simulink model "usrp_4t12r_heatmap"  (R2018a)
settings: Solver=VariableStepDiscrete  StartTime=0.0  StopTime=inf  RelTol=1e-3
undefined symbols (not defined in the file): fft2, gather, get, gpuArray, parula, psBcoor, psWcen, rfcaptureC2Fsim, Time, tsRamp, us
libraries: neural x14, visionanalysis x8, dspobslib x8, dspfdesign x7, dspstat3 x5, dspbuff3 x2, visionsinks x2, commsdrhw_v2 x1, visiontextngfix x1, dspvision x1, visiontransforms x1, dspsigops x1
(part 2 of 4)

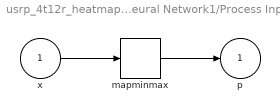
== system usrp_4t12r_heatmap/定位系统/定位模块/Pattern Recognition Neural Network1/Process Input 1 ==
  x : Inport  PortDimensions=627
      mask Display: e = 0.06;c1 = [120 230 180]/255;c2 = ([120 230 180]+0)/(256+128);c3 = ([120 230 180]+128)/(256+128);patch([0 1 1 0],[0 0 1 1],c1);patch([0 1 1 1-e 1-e 0+e],[0 0 1 1-e 0+e 0+e],c2);patch([0 0 1 1-e 0+e 0+e],[0 1 1 1-e 1-e 0+e],c3);plot([0 1 1 0 0],[0 0 1 1 0]);
  mapminmax : neural/Processing Functions/mapminmax  xmin=[0.183030532688018526821238651792;0.190861261961224687455640491862;0.194146917626080439678304401241;0.183721955574710132941262941131;0.201842690762400661652620215136;0.220412633155252224437248287359;0.210318465182484953812647177074;0.225823707454154809504132117581;0.243135323014785853512620406036;0.221810071164261130016726042413;0.218352813453565136603273799665;0.217860424693131021767200650174;0.211451016642378614163177985574;0.209356237294615388222496221715;0.205818369605545864464701821817;0.197728209339595090154872991661;0.190530847063016622877640315892;0.167795272037218085037224568623;0.144670324129353350395277288953;0.183030532688018526821238651792;0.190861261961224687455640491862;0.194146917626080439678304401241;0.183721955574710132941262941131;0.201842690762400661652620215136;0.220412633155252224437248287359;0.210318465182484953812647177074;0.225823707454154809504132117581;0.243135323014785853512620406036;0.221810071164261130016726042413;0.218352813453565136603273799665;0.217860424693131021767200650174;0.211451016642378614163177985574;0.209356237294615388222496221715;0.205818369605545864464701821817;0.197728209339595090154872991661;0.190530847063016622877640315892;0.167795272037218085037224568623;0.144670324129353350395277288953;0.183030532688018526821238651792;0.190861261961224687455640491862;0.194146917626080439678304401241;0.183721955574710132941262941131;0.201842690762400661652620215136;0.220412633155252224437248287359;0.210318465182484953812647177074;0.225823707454154809504132117581;0.243135323014785853512620406036;0.221810071164261130016726042413;0.218352813453565136603273799665;0.217860424693131021767200650174;0.211451016642378614163177985574;0.209356237294615388222496221715;0.205818369605545864464701821817;0.197728209339595090154872991661;0.190530847063016622877640315892;0.167795272037218085037224568623;0.144670324129353350395277288953;0.183030532688018526821238651792;0.190861261961224687455640491862;0.194146917626080439678304401241;0.183721955574710132941262941131;0.201842690762400661652620215136;0.220412633155252224437248287359;0.210318465182484953812647177074;0.225823707454154809504132117581;0.243135323014785853512620406036;0.221810071164261130016726042413;0.218352813453565136603273799665;0.217860424693131021767200650174;0.211451016642378614163177985574;0.209356237294615388222496221715;0.205818369605545864464701821817;0.197728209339595090154872991661;0.190530847063016622877640315892;0.167795272037218085037224568623;0.144670324129353350395277288953;0.188373791055123723792164014412;0.196433124862748803574064027089;0.194146917626080439678304401241;0.183721955574710132941262941131;0.201842690762400661652620215136;0.220412633155252224437248287359;0.210318465182484953812647177074;0.225823707454154809504132117581;0.243135323014785853512620406036;0.221810071164261130016726042413;0.218352813453565136603273799665;0.217860424693131021767200650174;0.211451016642378614163177985574;0.209356237294615388222496221715;0.205818369605545864464701821817;0.197728209339595090154872991661;0.190530847063016622877640315892;0.167795272037218085037224568623;0.144670324129353350395277288953;0.188373791055123723792164014412;0.196433124862748803574064027089;0.194146917626080439678304401241;0.183721955574710132941262941131;0.201842690762400661652620215136;0.220412633155252224437248287359;0.210318465182484953812647177074;0.225823707454154809504132117581;0.243135323014785853512620406036;0.221810071164261130016726042413;0.218352813453565136603273799665;0.217860424693131021767200650174;0.211451016642378614163177985574;0.209356237294615388222496221715;0.205818369605545864464701821817;0.197728209339595090154872991661;0.190530847063016622877640315892;0.167795272037218085037224568623;0.144670324129353350395277288953;0.197827438261914317907397276031;0.204571901720102755639629776852;0.194146917626080439678304401241;0.183721955574710132941262941131;0.201842690762400661652620215136;0.220412633155252224437248287359;0.216458347323125160910350928134 ...(+16650 chars)]  xmax=[1;0.957688668661197506359883391269;0.957956127733447404537514557887;1;0.996524641407459332853591149615;1;1;1;1;1;1;1;1;1;1;1;0.992949114404950594625631765666;0.983183728188606664843973703682;0.975467151452690028889946916024;1;0.960233553399059580613084108336;0.957956127733447404537514557887;1;0.996524641407459332853591149615;1;1;0.996308649645406885220211279375;1;1;1;0.99394380170718721334566225778;1;1;1;1;0.992949114404950594625631765666;0.983183728188606664843973703682;0.975467151452690028889946916024;1;0.960233553399059580613084108336;0.971339192350340052684032343677;1;0.996524641407459332853591149615;1;1;0.987208758234387806496101802622;0.996476557864772627404192917311;1;1;0.99394380170718721334566225778;1;1;0.996365674241340815164846844709;1;0.992949114404950594625631765666;0.983183728188606664843973703682;0.975467151452690028889946916024;1;0.960233553399059580613084108336;0.971339192350340052684032343677;1;1;1;1;0.987208758234387806496101802622;0.998269531990686354028241566994;1;1;0.99394380170718721334566225778;1;1;1;1;0.992949114404950594625631765666;0.983183728188606664843973703682;0.975467151452690028889946916024;0.992019539944344441728674155456;0.960233553399059580613084108336;0.971339192350340052684032343677;1;1;1;1;0.987208758234387806496101802622;0.998269531990686354028241566994;1;1;0.99394380170718721334566225778;1;1;1;1;0.992949114404950594625631765666;0.983183728188606664843973703682;0.975467151452690028889946916024;0.965464417572932775968297391955;0.952570447882058246591441275086;0.971339192350340052684032343677;1;1;1;1;0.976132306177093567178815192165;0.998269531990686354028241566994;1;0.984196482050718746137363268645;0.99394380170718721334566225778;1;1;1;1;0.992949114404950594625631765666;0.983183728188606664843973703682;0.975467151452690028889946916024;0.953175834974080649075744986476;0.932443563986340873128710882156;0.971339192350340052684032343677;1;1;1;1;0.976132306177093567178815192165;0.998269531990686354028241566994;1;0.984196482050718746137363268645;0.99394380170718721334566225778;1;1;1;1;0.992949114404950594625631765666;0.983183728188606664843973703682;0.975467151452690028889946916024;0.981027149358607908347096326906;1;0.978869445923384651209175899567;0.991702730309424129728768093628;1;1;1;0.980384429143986713128811061324;0.998269531990686354028241566994;1;0.984196482050718746137363268645;0.99394380170718721334566225778;1;1;1;1;0.992949114404950594625631765666;0.983183728188606664843973703682;0.975467151452690028889946916024;0.981027149358607908347096326906;1;0.978869445923384651209175899567;0.991702730309424129728768093628;1;1;1;0.980384429143986713128811061324;0.998269531990686354028241566994;1;0.984196482050718746137363268645;0.99394380170718721334566225778;1;1;1;1;0.992949114404950594625631765666;0.983183728188606664843973703682;0.975467151452690028889946916024;0.981027149358607908347096326906;1;0.978869445923384651209175899567;0.991702730309424129728768093628;1;1;1;0.980384429143986713128811061324;0.998269531990686354028241566994;1;0.984196482050718746137363268645;0.99394380170718721334566225778;1;1;1;1;0.992949114404950594625631765666;0.983183728188606664843973703682;0.975467151452690028889946916024;0.981027149358607908347096326906;1;0.978869445923384651209175899567;0.991702730309424129728768093628;1;1;1;0.980384429143986713128811061324;0.998269531990686354028241566994;1;0.984196482050718746137363268645;0.99394380170718721334566225778;1;1;1;1;0.992949114404950594625631765666;0.983183728188606664843973703682;0.975467151452690028889946916024;0.981027149358607908347096326906;1;0.978869445923384651209175899567;0.991702730309424129728768093628;1;1;1;0.980384429143986713128811061324;0.998269531990686354028241566994;1;0.998970019032386580271065668057;1;1;1;1;0.999424539007601864248897527432;0.992949114404950594625631765666;0.983183728188606664843973703682;0.975467151452690028889946916024;0.981027149358607908347096326906;1;0.978869445923384651209175899567;0.991702730309424129728768093628;1;1;1 ...(+8309 chars)]  ymin=-1  ymax=1
  p : Outport  PortDimensions=627
      mask Display: e = 0.06;c1 = [120 230 180]/255;c2 = ([120 230 180]+0)/(256+128);c3 = ([120 230 180]+128)/(256+128);patch([0 1 1 0],[0 0 1 1],c1);patch([0 1 1 1-e 1-e 0+e],[0 0 1 1-e 0+e 0+e],c2);patch([0 0 1 1-e 0+e 0+e],[0 1 1 1-e 1-e 0+e],c3);plot([0 1 1 0 0],[0 0 1 1 0]);
  wires:
  x/1 -> mapminmax/1
  mapminmax/1 -> p/1

== system usrp_4t12r_heatmap/定位系统/定位模块/Pattern Recognition Neural Network1/Process Output 1 ==
  a : Inport  PortDimensions=1
      mask Display: e = 0.06;c1 = [120 230 180]/255;c2 = ([120 230 180]+0)/(256+128);c3 = ([120 230 180]+128)/(256+128);patch([0 1 1 0],[0 0 1 1],c1);patch([0 1 1 1-e 1-e 0+e],[0 0 1 1-e 0+e 0+e],c2);patch([0 0 1 1-e 0+e 0+e],[0 1 1 1-e 1-e 0+e],c3);plot([0 1 1 0 0],[0 0 1 1 0]);
  y : Outport  PortDimensions=1
      mask Display: e = 0.06;c1 = [120 230 180]/255;c2 = ([120 230 180]+0)/(256+128);c3 = ([120 230 180]+128)/(256+128);patch([0 1 1 0],[0 0 1 1],c1);patch([0 1 1 1-e 1-e 0+e],[0 0 1 1-e 0+e 0+e],c2);patch([0 0 1 1-e 0+e 0+e],[0 1 1 1-e 1-e 0+e],c3);plot([0 1 1 0 0],[0 0 1 1 0]);
  wires:
  a/1 -> y/1

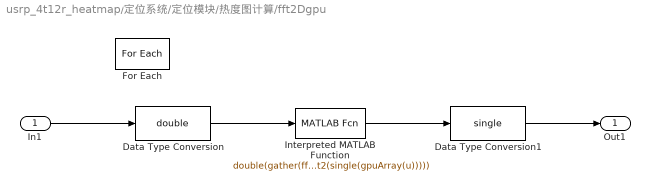
== system usrp_4t12r_heatmap/定位系统/定位模块/热度图计算/fft2Dgpu ==
  In1 : Inport  Partition=on  PartitionDimension=3  PartitionWidth=1  PartitionOffset=0
  Data Type Conversion : DataTypeConversion  OutDataTypeStr=double
  Data Type Conversion1 : DataTypeConversion  OutDataTypeStr=single
  For Each : ForEach  DisableCoverage=on  IndexMode=One-based
  Interpreted MATLAB Function : MATLABFcn  MATLABFcn=double(gather(fft2(single(gpuArray(u)))))  Output1D=off
  Out1 : Outport  ConcatenationDimension=3
  wires:
  In1/1 -> Data Type Conversion/1
  Interpreted MATLAB Function/1 -> Data Type Conversion1/1
  Data Type Conversion/1 -> Interpreted MATLAB Function/1
  Data Type Conversion1/1 -> Out1/1

== system usrp_4t12r_heatmap/定位系统/定位模块/Pattern Recognition Neural Network1/Layer 1/Delays 1 ==
  "p{1}" : Inport  PortDimensions=627
      mask Display: e = 0.06;c1 = [120 230 180]/255;c2 = ([120 230 180]+0)/(256+128);c3 = ([120 230 180]+128)/(256+128);patch([0 1 1 0],[0 0 1 1],c1);patch([0 1 1 1-e 1-e 0+e],[0 0 1 1-e 0+e 0+e],c2);patch([0 0 1 1-e 0+e 0+e],[0 1 1 1-e 1-e 0+e],c3);plot([0 1 1 0 0],[0 0 1 1 0]);
  mux : Mux  Inputs=1
      mask Display: e = 0.06;c1 = [120 150 230]/255;c2 = ([120 150 230]+0)/383;c3 = ([120 150 230]+128)/383;patch([0 1 1 0],[0 0 1 1],c1);patch([0 1 1 1-e 1-e 0+e],[0 0 1 1-e 0+e 0+e],c2);patch([0 0 1 1-e 0+e 0+e],[0 1 1 1-e 1-e 0+e],c3);plot([0 1 1 0 0],[0 0 1 1 0]);disp('Mux')
  "pd{1,1}" : Outport
      mask Display: e = 0.06;c1 = [120 230 180]/255;c2 = ([120 230 180]+0)/(256+128);c3 = ([120 230 180]+128)/(256+128);patch([0 1 1 0],[0 0 1 1],c1);patch([0 1 1 1-e 1-e 0+e],[0 0 1 1-e 0+e 0+e],c2);patch([0 0 1 1-e 0+e 0+e],[0 1 1 1-e 1-e 0+e],c3);plot([0 1 1 0 0],[0 0 1 1 0]);
  wires:
  "p{1}"/1 -> mux/1
  mux/1 -> "pd{1,1}"/1
